simulink model "PEArray_co_sim"  (R2021a)
settings: Solver=VariableStepAuto  StartTime=0.0  StopTime=15  RelTol=1e-3
undefined symbols (not defined in the file or in its folder): A, N
libraries: hdlBasic x164, xbsIndex_r4 x1, JTAGRuntimeCosim_r4 x1
(part 2 of 2)

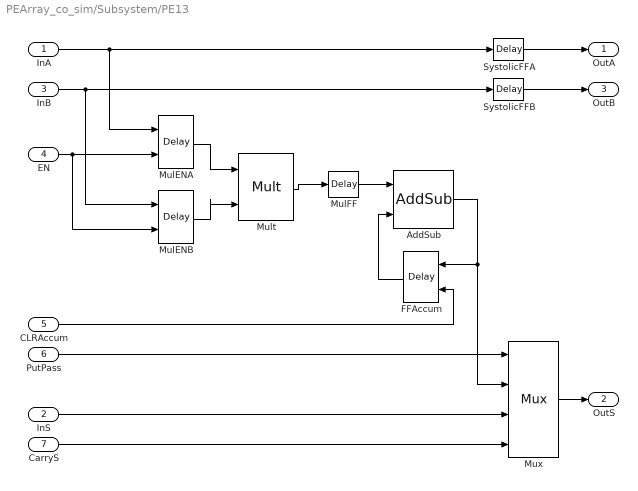
== system PEArray_co_sim/Subsystem/PE13 ==
  InA : Inport
  InS : Inport  Port=2
  InB : Inport  Port=3
  EN : Inport  Port=4
  CLRAccum : Inport  Port=5
  PutPass : Inport  Port=6
  CarryS : Inport  Port=7
  AddSub : hdlBasic/AddSub  mode=Addition  use_carryin=off  use_carryout=off  en=off  latency=0  precision=User Defined  arith_type="Signed  (2's comp)"  n_bits=16  bin_pt=10  quantization=Truncate  overflow=Wrap  use_behavioral_HDL=off  hw_selection=DSP48  pipelined=off  XmcBlockStatus=1  maskContainerNames=tabcontainer1  block_type=addsub  block_config=sysgen:Addsub_config
  FFAccum : hdlBasic/Delay  rst=on  en=off  latency=1  reg_retiming=off  XmcBlockStatus=1  maskContainerNames=group1  block_type=delay  block_config=sysgen:Delay_config
  MulENA : hdlBasic/Delay  rst=on  en=off  latency=1  reg_retiming=off  XmcBlockStatus=1  maskContainerNames=group1  block_type=delay  block_config=sysgen:Delay_config
  MulENB : hdlBasic/Delay  rst=on  en=off  latency=1  reg_retiming=off  XmcBlockStatus=1  maskContainerNames=group1  block_type=delay  block_config=sysgen:Delay_config
  MulFF : hdlBasic/Delay  rst=off  en=off  latency=1  reg_retiming=off  XmcBlockStatus=1  maskContainerNames=group1  block_type=delay  block_config=sysgen:Delay_config
  Mult : hdlBasic/Mult  precision=User Defined  arith_type="Signed  (2's comp)"  n_bits=16  bin_pt=10  quantization=Truncate  overflow=Wrap  en=off  latency=0  use_behavioral_HDL=off  opt=Speed  use_embedded=on  optimum_pipeline=off  pipeline=on  use_rpm=on  placement_style=Triangular  XmcBlockStatus=1  maskContainerNames=group1  block_type=mult  block_config=sysgen:Mult_config
  Mux : hdlBasic/Mux  inputs=2  en=on  latency=1  precision=Full  arith_type=Unsigned  n_bits=16  bin_pt=14  quantization=Truncate  overflow=Wrap  XmcBlockStatus=1  maskContainerNames=tabcontainer1  block_type=mux  block_config=sysgen:Mux_config
  SystolicFFA : hdlBasic/Delay  rst=off  en=off  latency=1  reg_retiming=off  XmcBlockStatus=1  maskContainerNames=group1  block_type=delay  block_config=sysgen:Delay_config
  SystolicFFB : hdlBasic/Delay  rst=off  en=off  latency=1  reg_retiming=off  XmcBlockStatus=1  maskContainerNames=group1  block_type=delay  block_config=sysgen:Delay_config
  OutA : Outport
  OutS : Outport  Port=2
  OutB : Outport  Port=3
  wires:
  Mult/1 -> MulFF/1
  MulFF/1 -> AddSub/1
  AddSub/1 -> Mux/2, FFAccum/1
  InB/1 -> MulENB/1, SystolicFFB/1
  InA/1 -> MulENA/1, SystolicFFA/1
  SystolicFFB/1 -> OutB/1
  SystolicFFA/1 -> OutA/1
  MulENA/1 -> Mult/1
  MulENB/1 -> Mult/2
  EN/1 -> MulENB/2, MulENA/2
  FFAccum/1 -> AddSub/2
  CLRAccum/1 -> FFAccum/2
  PutPass/1 -> Mux/1
  InS/1 -> Mux/3
  Mux/1 -> OutS/1
  CarryS/1 -> Mux/4

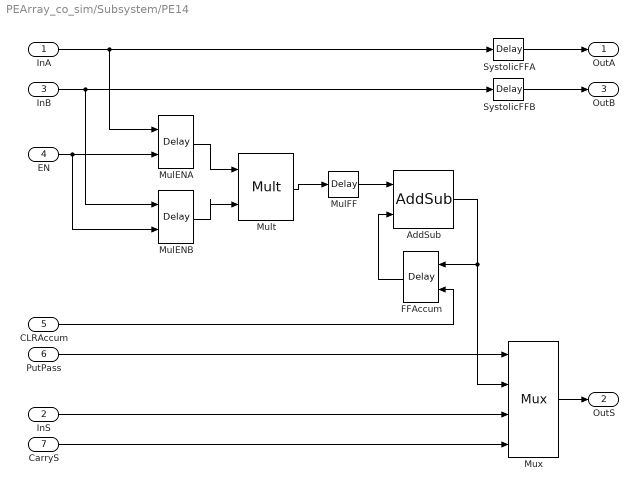
== system PEArray_co_sim/Subsystem/PE14 ==
  InA : Inport
  InS : Inport  Port=2
  InB : Inport  Port=3
  EN : Inport  Port=4
  CLRAccum : Inport  Port=5
  PutPass : Inport  Port=6
  CarryS : Inport  Port=7
  AddSub : hdlBasic/AddSub  mode=Addition  use_carryin=off  use_carryout=off  en=off  latency=0  precision=User Defined  arith_type="Signed  (2's comp)"  n_bits=16  bin_pt=10  quantization=Truncate  overflow=Wrap  use_behavioral_HDL=off  hw_selection=DSP48  pipelined=off  XmcBlockStatus=1  maskContainerNames=tabcontainer1  block_type=addsub  block_config=sysgen:Addsub_config
  FFAccum : hdlBasic/Delay  rst=on  en=off  latency=1  reg_retiming=off  XmcBlockStatus=1  maskContainerNames=group1  block_type=delay  block_config=sysgen:Delay_config
  MulENA : hdlBasic/Delay  rst=on  en=off  latency=1  reg_retiming=off  XmcBlockStatus=1  maskContainerNames=group1  block_type=delay  block_config=sysgen:Delay_config
  MulENB : hdlBasic/Delay  rst=on  en=off  latency=1  reg_retiming=off  XmcBlockStatus=1  maskContainerNames=group1  block_type=delay  block_config=sysgen:Delay_config
  MulFF : hdlBasic/Delay  rst=off  en=off  latency=1  reg_retiming=off  XmcBlockStatus=1  maskContainerNames=group1  block_type=delay  block_config=sysgen:Delay_config
  Mult : hdlBasic/Mult  precision=User Defined  arith_type="Signed  (2's comp)"  n_bits=16  bin_pt=10  quantization=Truncate  overflow=Wrap  en=off  latency=0  use_behavioral_HDL=off  opt=Speed  use_embedded=on  optimum_pipeline=off  pipeline=on  use_rpm=on  placement_style=Triangular  XmcBlockStatus=1  maskContainerNames=group1  block_type=mult  block_config=sysgen:Mult_config
  Mux : hdlBasic/Mux  inputs=2  en=on  latency=1  precision=Full  arith_type=Unsigned  n_bits=16  bin_pt=14  quantization=Truncate  overflow=Wrap  XmcBlockStatus=1  maskContainerNames=tabcontainer1  block_type=mux  block_config=sysgen:Mux_config
  SystolicFFA : hdlBasic/Delay  rst=off  en=off  latency=1  reg_retiming=off  XmcBlockStatus=1  maskContainerNames=group1  block_type=delay  block_config=sysgen:Delay_config
  SystolicFFB : hdlBasic/Delay  rst=off  en=off  latency=1  reg_retiming=off  XmcBlockStatus=1  maskContainerNames=group1  block_type=delay  block_config=sysgen:Delay_config
  OutA : Outport
  OutS : Outport  Port=2
  OutB : Outport  Port=3
  wires:
  Mult/1 -> MulFF/1
  MulFF/1 -> AddSub/1
  AddSub/1 -> Mux/2, FFAccum/1
  InB/1 -> MulENB/1, SystolicFFB/1
  InA/1 -> MulENA/1, SystolicFFA/1
  SystolicFFB/1 -> OutB/1
  SystolicFFA/1 -> OutA/1
  MulENA/1 -> Mult/1
  MulENB/1 -> Mult/2
  EN/1 -> MulENB/2, MulENA/2
  FFAccum/1 -> AddSub/2
  CLRAccum/1 -> FFAccum/2
  PutPass/1 -> Mux/1
  InS/1 -> Mux/3
  Mux/1 -> OutS/1
  CarryS/1 -> Mux/4

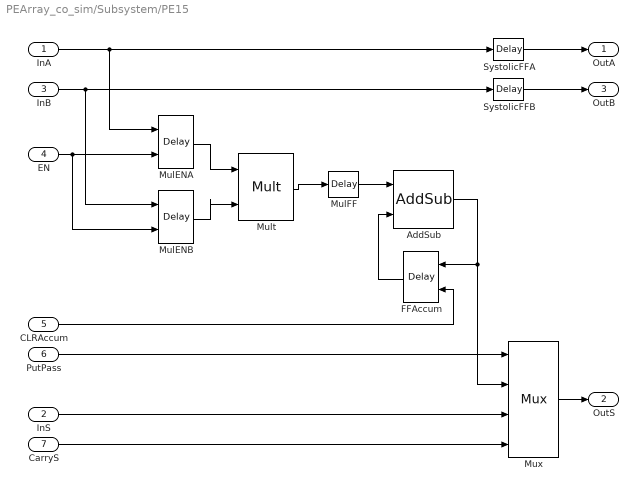
== system PEArray_co_sim/Subsystem/PE15 ==
  InA : Inport
  InS : Inport  Port=2
  InB : Inport  Port=3
  EN : Inport  Port=4
  CLRAccum : Inport  Port=5
  PutPass : Inport  Port=6
  CarryS : Inport  Port=7
  AddSub : hdlBasic/AddSub  mode=Addition  use_carryin=off  use_carryout=off  en=off  latency=0  precision=User Defined  arith_type="Signed  (2's comp)"  n_bits=16  bin_pt=10  quantization=Truncate  overflow=Wrap  use_behavioral_HDL=off  hw_selection=DSP48  pipelined=off  XmcBlockStatus=1  maskContainerNames=tabcontainer1  block_type=addsub  block_config=sysgen:Addsub_config
  FFAccum : hdlBasic/Delay  rst=on  en=off  latency=1  reg_retiming=off  XmcBlockStatus=1  maskContainerNames=group1  block_type=delay  block_config=sysgen:Delay_config
  MulENA : hdlBasic/Delay  rst=on  en=off  latency=1  reg_retiming=off  XmcBlockStatus=1  maskContainerNames=group1  block_type=delay  block_config=sysgen:Delay_config
  MulENB : hdlBasic/Delay  rst=on  en=off  latency=1  reg_retiming=off  XmcBlockStatus=1  maskContainerNames=group1  block_type=delay  block_config=sysgen:Delay_config
  MulFF : hdlBasic/Delay  rst=off  en=off  latency=1  reg_retiming=off  XmcBlockStatus=1  maskContainerNames=group1  block_type=delay  block_config=sysgen:Delay_config
  Mult : hdlBasic/Mult  precision=User Defined  arith_type="Signed  (2's comp)"  n_bits=16  bin_pt=10  quantization=Truncate  overflow=Wrap  en=off  latency=0  use_behavioral_HDL=off  opt=Speed  use_embedded=on  optimum_pipeline=off  pipeline=on  use_rpm=on  placement_style=Triangular  XmcBlockStatus=1  maskContainerNames=group1  block_type=mult  block_config=sysgen:Mult_config
  Mux : hdlBasic/Mux  inputs=2  en=on  latency=1  precision=Full  arith_type=Unsigned  n_bits=16  bin_pt=14  quantization=Truncate  overflow=Wrap  XmcBlockStatus=1  maskContainerNames=tabcontainer1  block_type=mux  block_config=sysgen:Mux_config
  SystolicFFA : hdlBasic/Delay  rst=off  en=off  latency=1  reg_retiming=off  XmcBlockStatus=1  maskContainerNames=group1  block_type=delay  block_config=sysgen:Delay_config
  SystolicFFB : hdlBasic/Delay  rst=off  en=off  latency=1  reg_retiming=off  XmcBlockStatus=1  maskContainerNames=group1  block_type=delay  block_config=sysgen:Delay_config
  OutA : Outport
  OutS : Outport  Port=2
  OutB : Outport  Port=3
  wires:
  Mult/1 -> MulFF/1
  MulFF/1 -> AddSub/1
  AddSub/1 -> Mux/2, FFAccum/1
  InB/1 -> MulENB/1, SystolicFFB/1
  InA/1 -> MulENA/1, SystolicFFA/1
  SystolicFFB/1 -> OutB/1
  SystolicFFA/1 -> OutA/1
  MulENA/1 -> Mult/1
  MulENB/1 -> Mult/2
  EN/1 -> MulENB/2, MulENA/2
  FFAccum/1 -> AddSub/2
  CLRAccum/1 -> FFAccum/2
  PutPass/1 -> Mux/1
  InS/1 -> Mux/3
  Mux/1 -> OutS/1
  CarryS/1 -> Mux/4

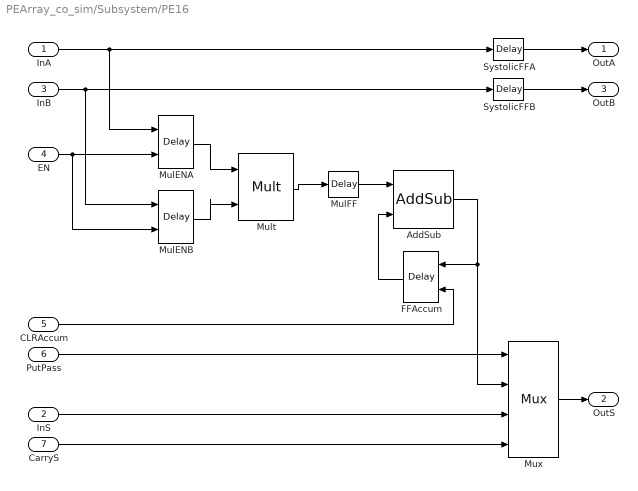
== system PEArray_co_sim/Subsystem/PE16 ==
  InA : Inport
  InS : Inport  Port=2
  InB : Inport  Port=3
  EN : Inport  Port=4
  CLRAccum : Inport  Port=5
  PutPass : Inport  Port=6
  CarryS : Inport  Port=7
  AddSub : hdlBasic/AddSub  mode=Addition  use_carryin=off  use_carryout=off  en=off  latency=0  precision=User Defined  arith_type="Signed  (2's comp)"  n_bits=16  bin_pt=10  quantization=Truncate  overflow=Wrap  use_behavioral_HDL=off  hw_selection=DSP48  pipelined=off  XmcBlockStatus=1  maskContainerNames=tabcontainer1  block_type=addsub  block_config=sysgen:Addsub_config
  FFAccum : hdlBasic/Delay  rst=on  en=off  latency=1  reg_retiming=off  XmcBlockStatus=1  maskContainerNames=group1  block_type=delay  block_config=sysgen:Delay_config
  MulENA : hdlBasic/Delay  rst=on  en=off  latency=1  reg_retiming=off  XmcBlockStatus=1  maskContainerNames=group1  block_type=delay  block_config=sysgen:Delay_config
  MulENB : hdlBasic/Delay  rst=on  en=off  latency=1  reg_retiming=off  XmcBlockStatus=1  maskContainerNames=group1  block_type=delay  block_config=sysgen:Delay_config
  MulFF : hdlBasic/Delay  rst=off  en=off  latency=1  reg_retiming=off  XmcBlockStatus=1  maskContainerNames=group1  block_type=delay  block_config=sysgen:Delay_config
  Mult : hdlBasic/Mult  precision=User Defined  arith_type="Signed  (2's comp)"  n_bits=16  bin_pt=10  quantization=Truncate  overflow=Wrap  en=off  latency=0  use_behavioral_HDL=off  opt=Speed  use_embedded=on  optimum_pipeline=off  pipeline=on  use_rpm=on  placement_style=Triangular  XmcBlockStatus=1  maskContainerNames=group1  block_type=mult  block_config=sysgen:Mult_config
  Mux : hdlBasic/Mux  inputs=2  en=on  latency=1  precision=Full  arith_type=Unsigned  n_bits=16  bin_pt=14  quantization=Truncate  overflow=Wrap  XmcBlockStatus=1  maskContainerNames=tabcontainer1  block_type=mux  block_config=sysgen:Mux_config
  SystolicFFA : hdlBasic/Delay  rst=off  en=off  latency=1  reg_retiming=off  XmcBlockStatus=1  maskContainerNames=group1  block_type=delay  block_config=sysgen:Delay_config
  SystolicFFB : hdlBasic/Delay  rst=off  en=off  latency=1  reg_retiming=off  XmcBlockStatus=1  maskContainerNames=group1  block_type=delay  block_config=sysgen:Delay_config
  OutA : Outport
  OutS : Outport  Port=2
  OutB : Outport  Port=3
  wires:
  Mult/1 -> MulFF/1
  MulFF/1 -> AddSub/1
  AddSub/1 -> Mux/2, FFAccum/1
  InB/1 -> MulENB/1, SystolicFFB/1
  InA/1 -> MulENA/1, SystolicFFA/1
  SystolicFFB/1 -> OutB/1
  SystolicFFA/1 -> OutA/1
  MulENA/1 -> Mult/1
  MulENB/1 -> Mult/2
  EN/1 -> MulENB/2, MulENA/2
  FFAccum/1 -> AddSub/2
  CLRAccum/1 -> FFAccum/2
  PutPass/1 -> Mux/1
  InS/1 -> Mux/3
  Mux/1 -> OutS/1
  CarryS/1 -> Mux/4

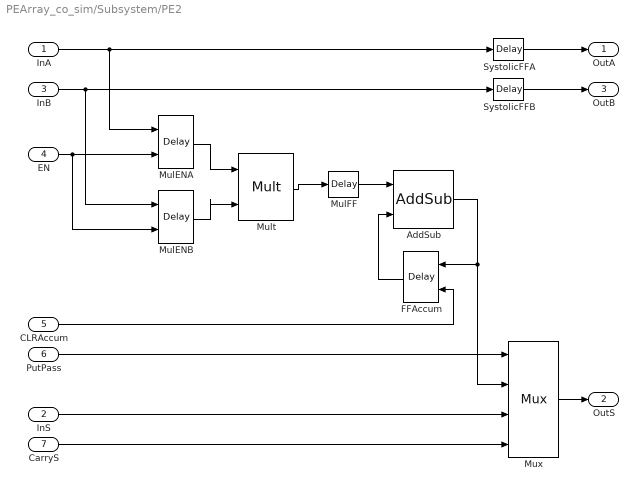
== system PEArray_co_sim/Subsystem/PE2 ==
  InA : Inport
  InS : Inport  Port=2
  InB : Inport  Port=3
  EN : Inport  Port=4
  CLRAccum : Inport  Port=5
  PutPass : Inport  Port=6
  CarryS : Inport  Port=7
  AddSub : hdlBasic/AddSub  mode=Addition  use_carryin=off  use_carryout=off  en=off  latency=0  precision=User Defined  arith_type="Signed  (2's comp)"  n_bits=16  bin_pt=10  quantization=Truncate  overflow=Wrap  use_behavioral_HDL=off  hw_selection=DSP48  pipelined=off  XmcBlockStatus=1  maskContainerNames=tabcontainer1  block_type=addsub  block_config=sysgen:Addsub_config
  FFAccum : hdlBasic/Delay  rst=on  en=off  latency=1  reg_retiming=off  XmcBlockStatus=1  maskContainerNames=group1  block_type=delay  block_config=sysgen:Delay_config
  MulENA : hdlBasic/Delay  rst=on  en=off  latency=1  reg_retiming=off  XmcBlockStatus=1  maskContainerNames=group1  block_type=delay  block_config=sysgen:Delay_config
  MulENB : hdlBasic/Delay  rst=on  en=off  latency=1  reg_retiming=off  XmcBlockStatus=1  maskContainerNames=group1  block_type=delay  block_config=sysgen:Delay_config
  MulFF : hdlBasic/Delay  rst=off  en=off  latency=1  reg_retiming=off  XmcBlockStatus=1  maskContainerNames=group1  block_type=delay  block_config=sysgen:Delay_config
  Mult : hdlBasic/Mult  precision=User Defined  arith_type="Signed  (2's comp)"  n_bits=16  bin_pt=10  quantization=Truncate  overflow=Wrap  en=off  latency=0  use_behavioral_HDL=off  opt=Speed  use_embedded=on  optimum_pipeline=off  pipeline=on  use_rpm=on  placement_style=Triangular  XmcBlockStatus=1  maskContainerNames=group1  block_type=mult  block_config=sysgen:Mult_config
  Mux : hdlBasic/Mux  inputs=2  en=on  latency=1  precision=Full  arith_type=Unsigned  n_bits=16  bin_pt=14  quantization=Truncate  overflow=Wrap  XmcBlockStatus=1  maskContainerNames=tabcontainer1  block_type=mux  block_config=sysgen:Mux_config
  SystolicFFA : hdlBasic/Delay  rst=off  en=off  latency=1  reg_retiming=off  XmcBlockStatus=1  maskContainerNames=group1  block_type=delay  block_config=sysgen:Delay_config
  SystolicFFB : hdlBasic/Delay  rst=off  en=off  latency=1  reg_retiming=off  XmcBlockStatus=1  maskContainerNames=group1  block_type=delay  block_config=sysgen:Delay_config
  OutA : Outport
  OutS : Outport  Port=2
  OutB : Outport  Port=3
  wires:
  Mult/1 -> MulFF/1
  MulFF/1 -> AddSub/1
  AddSub/1 -> Mux/2, FFAccum/1
  InB/1 -> MulENB/1, SystolicFFB/1
  InA/1 -> MulENA/1, SystolicFFA/1
  SystolicFFB/1 -> OutB/1
  SystolicFFA/1 -> OutA/1
  MulENA/1 -> Mult/1
  MulENB/1 -> Mult/2
  EN/1 -> MulENB/2, MulENA/2
  FFAccum/1 -> AddSub/2
  CLRAccum/1 -> FFAccum/2
  PutPass/1 -> Mux/1
  InS/1 -> Mux/3
  Mux/1 -> OutS/1
  CarryS/1 -> Mux/4

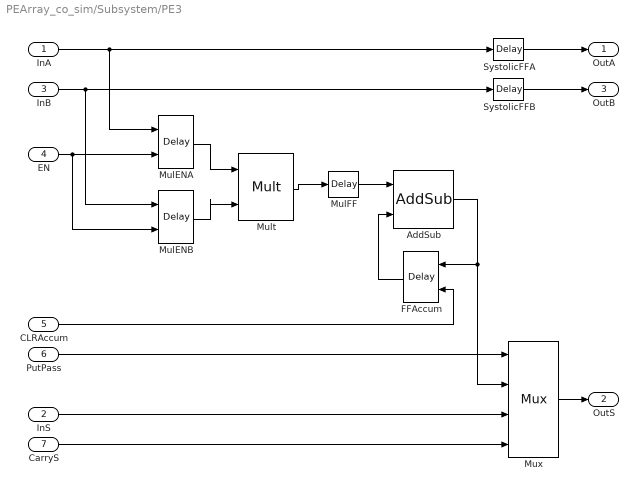
== system PEArray_co_sim/Subsystem/PE3 ==
  InA : Inport
  InS : Inport  Port=2
  InB : Inport  Port=3
  EN : Inport  Port=4
  CLRAccum : Inport  Port=5
  PutPass : Inport  Port=6
  CarryS : Inport  Port=7
  AddSub : hdlBasic/AddSub  mode=Addition  use_carryin=off  use_carryout=off  en=off  latency=0  precision=User Defined  arith_type="Signed  (2's comp)"  n_bits=16  bin_pt=10  quantization=Truncate  overflow=Wrap  use_behavioral_HDL=off  hw_selection=DSP48  pipelined=off  XmcBlockStatus=1  maskContainerNames=tabcontainer1  block_type=addsub  block_config=sysgen:Addsub_config
  FFAccum : hdlBasic/Delay  rst=on  en=off  latency=1  reg_retiming=off  XmcBlockStatus=1  maskContainerNames=group1  block_type=delay  block_config=sysgen:Delay_config
  MulENA : hdlBasic/Delay  rst=on  en=off  latency=1  reg_retiming=off  XmcBlockStatus=1  maskContainerNames=group1  block_type=delay  block_config=sysgen:Delay_config
  MulENB : hdlBasic/Delay  rst=on  en=off  latency=1  reg_retiming=off  XmcBlockStatus=1  maskContainerNames=group1  block_type=delay  block_config=sysgen:Delay_config
  MulFF : hdlBasic/Delay  rst=off  en=off  latency=1  reg_retiming=off  XmcBlockStatus=1  maskContainerNames=group1  block_type=delay  block_config=sysgen:Delay_config
  Mult : hdlBasic/Mult  precision=User Defined  arith_type="Signed  (2's comp)"  n_bits=16  bin_pt=10  quantization=Truncate  overflow=Wrap  en=off  latency=0  use_behavioral_HDL=off  opt=Speed  use_embedded=on  optimum_pipeline=off  pipeline=on  use_rpm=on  placement_style=Triangular  XmcBlockStatus=1  maskContainerNames=group1  block_type=mult  block_config=sysgen:Mult_config
  Mux : hdlBasic/Mux  inputs=2  en=on  latency=1  precision=Full  arith_type=Unsigned  n_bits=16  bin_pt=14  quantization=Truncate  overflow=Wrap  XmcBlockStatus=1  maskContainerNames=tabcontainer1  block_type=mux  block_config=sysgen:Mux_config
  SystolicFFA : hdlBasic/Delay  rst=off  en=off  latency=1  reg_retiming=off  XmcBlockStatus=1  maskContainerNames=group1  block_type=delay  block_config=sysgen:Delay_config
  SystolicFFB : hdlBasic/Delay  rst=off  en=off  latency=1  reg_retiming=off  XmcBlockStatus=1  maskContainerNames=group1  block_type=delay  block_config=sysgen:Delay_config
  OutA : Outport
  OutS : Outport  Port=2
  OutB : Outport  Port=3
  wires:
  Mult/1 -> MulFF/1
  MulFF/1 -> AddSub/1
  AddSub/1 -> Mux/2, FFAccum/1
  InB/1 -> MulENB/1, SystolicFFB/1
  InA/1 -> MulENA/1, SystolicFFA/1
  SystolicFFB/1 -> OutB/1
  SystolicFFA/1 -> OutA/1
  MulENA/1 -> Mult/1
  MulENB/1 -> Mult/2
  EN/1 -> MulENB/2, MulENA/2
  FFAccum/1 -> AddSub/2
  CLRAccum/1 -> FFAccum/2
  PutPass/1 -> Mux/1
  InS/1 -> Mux/3
  Mux/1 -> OutS/1
  CarryS/1 -> Mux/4

== system PEArray_co_sim/Subsystem/PE4 ==
  InA : Inport
  InS : Inport  Port=2
  InB : Inport  Port=3
  EN : Inport  Port=4
  CLRAccum : Inport  Port=5
  PutPass : Inport  Port=6
  CarryS : Inport  Port=7
  AddSub : hdlBasic/AddSub  mode=Addition  use_carryin=off  use_carryout=off  en=off  latency=0  precision=User Defined  arith_type="Signed  (2's comp)"  n_bits=16  bin_pt=10  quantization=Truncate  overflow=Wrap  use_behavioral_HDL=off  hw_selection=DSP48  pipelined=off  XmcBlockStatus=1  maskContainerNames=tabcontainer1  block_type=addsub  block_config=sysgen:Addsub_config
  FFAccum : hdlBasic/Delay  rst=on  en=off  latency=1  reg_retiming=off  XmcBlockStatus=1  maskContainerNames=group1  block_type=delay  block_config=sysgen:Delay_config
  MulENA : hdlBasic/Delay  rst=on  en=off  latency=1  reg_retiming=off  XmcBlockStatus=1  maskContainerNames=group1  block_type=delay  block_config=sysgen:Delay_config
  MulENB : hdlBasic/Delay  rst=on  en=off  latency=1  reg_retiming=off  XmcBlockStatus=1  maskContainerNames=group1  block_type=delay  block_config=sysgen:Delay_config
  MulFF : hdlBasic/Delay  rst=off  en=off  latency=1  reg_retiming=off  XmcBlockStatus=1  maskContainerNames=group1  block_type=delay  block_config=sysgen:Delay_config
  Mult : hdlBasic/Mult  precision=User Defined  arith_type="Signed  (2's comp)"  n_bits=16  bin_pt=10  quantization=Truncate  overflow=Wrap  en=off  latency=0  use_behavioral_HDL=off  opt=Speed  use_embedded=on  optimum_pipeline=off  pipeline=on  use_rpm=on  placement_style=Triangular  XmcBlockStatus=1  maskContainerNames=group1  block_type=mult  block_config=sysgen:Mult_config
  Mux : hdlBasic/Mux  inputs=2  en=on  latency=1  precision=Full  arith_type=Unsigned  n_bits=16  bin_pt=14  quantization=Truncate  overflow=Wrap  XmcBlockStatus=1  maskContainerNames=tabcontainer1  block_type=mux  block_config=sysgen:Mux_config
  SystolicFFA : hdlBasic/Delay  rst=off  en=off  latency=1  reg_retiming=off  XmcBlockStatus=1  maskContainerNames=group1  block_type=delay  block_config=sysgen:Delay_config
  SystolicFFB : hdlBasic/Delay  rst=off  en=off  latency=1  reg_retiming=off  XmcBlockStatus=1  maskContainerNames=group1  block_type=delay  block_config=sysgen:Delay_config
  OutA : Outport
  OutS : Outport  Port=2
  OutB : Outport  Port=3
  wires:
  Mult/1 -> MulFF/1
  MulFF/1 -> AddSub/1
  AddSub/1 -> Mux/2, FFAccum/1
  InB/1 -> MulENB/1, SystolicFFB/1
  InA/1 -> MulENA/1, SystolicFFA/1
  SystolicFFB/1 -> OutB/1
  SystolicFFA/1 -> OutA/1
  MulENA/1 -> Mult/1
  MulENB/1 -> Mult/2
  EN/1 -> MulENB/2, MulENA/2
  FFAccum/1 -> AddSub/2
  CLRAccum/1 -> FFAccum/2
  PutPass/1 -> Mux/1
  InS/1 -> Mux/3
  Mux/1 -> OutS/1
  CarryS/1 -> Mux/4

== system PEArray_co_sim/Subsystem/PE5 ==
  InA : Inport
  InS : Inport  Port=2
  InB : Inport  Port=3
  EN : Inport  Port=4
  CLRAccum : Inport  Port=5
  PutPass : Inport  Port=6
  CarryS : Inport  Port=7
  AddSub : hdlBasic/AddSub  mode=Addition  use_carryin=off  use_carryout=off  en=off  latency=0  precision=User Defined  arith_type="Signed  (2's comp)"  n_bits=16  bin_pt=10  quantization=Truncate  overflow=Wrap  use_behavioral_HDL=off  hw_selection=DSP48  pipelined=off  XmcBlockStatus=1  maskContainerNames=tabcontainer1  block_type=addsub  block_config=sysgen:Addsub_config
  FFAccum : hdlBasic/Delay  rst=on  en=off  latency=1  reg_retiming=off  XmcBlockStatus=1  maskContainerNames=group1  block_type=delay  block_config=sysgen:Delay_config
  MulENA : hdlBasic/Delay  rst=on  en=off  latency=1  reg_retiming=off  XmcBlockStatus=1  maskContainerNames=group1  block_type=delay  block_config=sysgen:Delay_config
  MulENB : hdlBasic/Delay  rst=on  en=off  latency=1  reg_retiming=off  XmcBlockStatus=1  maskContainerNames=group1  block_type=delay  block_config=sysgen:Delay_config
  MulFF : hdlBasic/Delay  rst=off  en=off  latency=1  reg_retiming=off  XmcBlockStatus=1  maskContainerNames=group1  block_type=delay  block_config=sysgen:Delay_config
  Mult : hdlBasic/Mult  precision=User Defined  arith_type="Signed  (2's comp)"  n_bits=16  bin_pt=10  quantization=Truncate  overflow=Wrap  en=off  latency=0  use_behavioral_HDL=off  opt=Speed  use_embedded=on  optimum_pipeline=off  pipeline=on  use_rpm=on  placement_style=Triangular  XmcBlockStatus=1  maskContainerNames=group1  block_type=mult  block_config=sysgen:Mult_config
  Mux : hdlBasic/Mux  inputs=2  en=on  latency=1  precision=Full  arith_type=Unsigned  n_bits=16  bin_pt=14  quantization=Truncate  overflow=Wrap  XmcBlockStatus=1  maskContainerNames=tabcontainer1  block_type=mux  block_config=sysgen:Mux_config
  SystolicFFA : hdlBasic/Delay  rst=off  en=off  latency=1  reg_retiming=off  XmcBlockStatus=1  maskContainerNames=group1  block_type=delay  block_config=sysgen:Delay_config
  SystolicFFB : hdlBasic/Delay  rst=off  en=off  latency=1  reg_retiming=off  XmcBlockStatus=1  maskContainerNames=group1  block_type=delay  block_config=sysgen:Delay_config
  OutA : Outport
  OutS : Outport  Port=2
  OutB : Outport  Port=3
  wires:
  Mult/1 -> MulFF/1
  MulFF/1 -> AddSub/1
  AddSub/1 -> Mux/2, FFAccum/1
  InB/1 -> MulENB/1, SystolicFFB/1
  InA/1 -> MulENA/1, SystolicFFA/1
  SystolicFFB/1 -> OutB/1
  SystolicFFA/1 -> OutA/1
  MulENA/1 -> Mult/1
  MulENB/1 -> Mult/2
  EN/1 -> MulENB/2, MulENA/2
  FFAccum/1 -> AddSub/2
  CLRAccum/1 -> FFAccum/2
  PutPass/1 -> Mux/1
  InS/1 -> Mux/3
  Mux/1 -> OutS/1
  CarryS/1 -> Mux/4

== system PEArray_co_sim/Subsystem/PE6 ==
  InA : Inport
  InS : Inport  Port=2
  InB : Inport  Port=3
  EN : Inport  Port=4
  CLRAccum : Inport  Port=5
  PutPass : Inport  Port=6
  CarryS : Inport  Port=7
  AddSub : hdlBasic/AddSub  mode=Addition  use_carryin=off  use_carryout=off  en=off  latency=0  precision=User Defined  arith_type="Signed  (2's comp)"  n_bits=16  bin_pt=10  quantization=Truncate  overflow=Wrap  use_behavioral_HDL=off  hw_selection=DSP48  pipelined=off  XmcBlockStatus=1  maskContainerNames=tabcontainer1  block_type=addsub  block_config=sysgen:Addsub_config
  FFAccum : hdlBasic/Delay  rst=on  en=off  latency=1  reg_retiming=off  XmcBlockStatus=1  maskContainerNames=group1  block_type=delay  block_config=sysgen:Delay_config
  MulENA : hdlBasic/Delay  rst=on  en=off  latency=1  reg_retiming=off  XmcBlockStatus=1  maskContainerNames=group1  block_type=delay  block_config=sysgen:Delay_config
  MulENB : hdlBasic/Delay  rst=on  en=off  latency=1  reg_retiming=off  XmcBlockStatus=1  maskContainerNames=group1  block_type=delay  block_config=sysgen:Delay_config
  MulFF : hdlBasic/Delay  rst=off  en=off  latency=1  reg_retiming=off  XmcBlockStatus=1  maskContainerNames=group1  block_type=delay  block_config=sysgen:Delay_config
  Mult : hdlBasic/Mult  precision=User Defined  arith_type="Signed  (2's comp)"  n_bits=16  bin_pt=10  quantization=Truncate  overflow=Wrap  en=off  latency=0  use_behavioral_HDL=off  opt=Speed  use_embedded=on  optimum_pipeline=off  pipeline=on  use_rpm=on  placement_style=Triangular  XmcBlockStatus=1  maskContainerNames=group1  block_type=mult  block_config=sysgen:Mult_config
  Mux : hdlBasic/Mux  inputs=2  en=on  latency=1  precision=Full  arith_type=Unsigned  n_bits=16  bin_pt=14  quantization=Truncate  overflow=Wrap  XmcBlockStatus=1  maskContainerNames=tabcontainer1  block_type=mux  block_config=sysgen:Mux_config
  SystolicFFA : hdlBasic/Delay  rst=off  en=off  latency=1  reg_retiming=off  XmcBlockStatus=1  maskContainerNames=group1  block_type=delay  block_config=sysgen:Delay_config
  SystolicFFB : hdlBasic/Delay  rst=off  en=off  latency=1  reg_retiming=off  XmcBlockStatus=1  maskContainerNames=group1  block_type=delay  block_config=sysgen:Delay_config
  OutA : Outport
  OutS : Outport  Port=2
  OutB : Outport  Port=3
  wires:
  Mult/1 -> MulFF/1
  MulFF/1 -> AddSub/1
  AddSub/1 -> Mux/2, FFAccum/1
  InB/1 -> MulENB/1, SystolicFFB/1
  InA/1 -> MulENA/1, SystolicFFA/1
  SystolicFFB/1 -> OutB/1
  SystolicFFA/1 -> OutA/1
  MulENA/1 -> Mult/1
  MulENB/1 -> Mult/2
  EN/1 -> MulENB/2, MulENA/2
  FFAccum/1 -> AddSub/2
  CLRAccum/1 -> FFAccum/2
  PutPass/1 -> Mux/1
  InS/1 -> Mux/3
  Mux/1 -> OutS/1
  CarryS/1 -> Mux/4

== system PEArray_co_sim/Subsystem/PE7 ==
  InA : Inport
  InS : Inport  Port=2
  InB : Inport  Port=3
  EN : Inport  Port=4
  CLRAccum : Inport  Port=5
  PutPass : Inport  Port=6
  CarryS : Inport  Port=7
  AddSub : hdlBasic/AddSub  mode=Addition  use_carryin=off  use_carryout=off  en=off  latency=0  precision=User Defined  arith_type="Signed  (2's comp)"  n_bits=16  bin_pt=10  quantization=Truncate  overflow=Wrap  use_behavioral_HDL=off  hw_selection=DSP48  pipelined=off  XmcBlockStatus=1  maskContainerNames=tabcontainer1  block_type=addsub  block_config=sysgen:Addsub_config
  FFAccum : hdlBasic/Delay  rst=on  en=off  latency=1  reg_retiming=off  XmcBlockStatus=1  maskContainerNames=group1  block_type=delay  block_config=sysgen:Delay_config
  MulENA : hdlBasic/Delay  rst=on  en=off  latency=1  reg_retiming=off  XmcBlockStatus=1  maskContainerNames=group1  block_type=delay  block_config=sysgen:Delay_config
  MulENB : hdlBasic/Delay  rst=on  en=off  latency=1  reg_retiming=off  XmcBlockStatus=1  maskContainerNames=group1  block_type=delay  block_config=sysgen:Delay_config
  MulFF : hdlBasic/Delay  rst=off  en=off  latency=1  reg_retiming=off  XmcBlockStatus=1  maskContainerNames=group1  block_type=delay  block_config=sysgen:Delay_config
  Mult : hdlBasic/Mult  precision=User Defined  arith_type="Signed  (2's comp)"  n_bits=16  bin_pt=10  quantization=Truncate  overflow=Wrap  en=off  latency=0  use_behavioral_HDL=off  opt=Speed  use_embedded=on  optimum_pipeline=off  pipeline=on  use_rpm=on  placement_style=Triangular  XmcBlockStatus=1  maskContainerNames=group1  block_type=mult  block_config=sysgen:Mult_config
  Mux : hdlBasic/Mux  inputs=2  en=on  latency=1  precision=Full  arith_type=Unsigned  n_bits=16  bin_pt=14  quantization=Truncate  overflow=Wrap  XmcBlockStatus=1  maskContainerNames=tabcontainer1  block_type=mux  block_config=sysgen:Mux_config
  SystolicFFA : hdlBasic/Delay  rst=off  en=off  latency=1  reg_retiming=off  XmcBlockStatus=1  maskContainerNames=group1  block_type=delay  block_config=sysgen:Delay_config
  SystolicFFB : hdlBasic/Delay  rst=off  en=off  latency=1  reg_retiming=off  XmcBlockStatus=1  maskContainerNames=group1  block_type=delay  block_config=sysgen:Delay_config
  OutA : Outport
  OutS : Outport  Port=2
  OutB : Outport  Port=3
  wires:
  Mult/1 -> MulFF/1
  MulFF/1 -> AddSub/1
  AddSub/1 -> Mux/2, FFAccum/1
  InB/1 -> MulENB/1, SystolicFFB/1
  InA/1 -> MulENA/1, SystolicFFA/1
  SystolicFFB/1 -> OutB/1
  SystolicFFA/1 -> OutA/1
  MulENA/1 -> Mult/1
  MulENB/1 -> Mult/2
  EN/1 -> MulENB/2, MulENA/2
  FFAccum/1 -> AddSub/2
  CLRAccum/1 -> FFAccum/2
  PutPass/1 -> Mux/1
  InS/1 -> Mux/3
  Mux/1 -> OutS/1
  CarryS/1 -> Mux/4

== system PEArray_co_sim/Subsystem/PE8 ==
  InA : Inport
  InS : Inport  Port=2
  InB : Inport  Port=3
  EN : Inport  Port=4
  CLRAccum : Inport  Port=5
  PutPass : Inport  Port=6
  CarryS : Inport  Port=7
  AddSub : hdlBasic/AddSub  mode=Addition  use_carryin=off  use_carryout=off  en=off  latency=0  precision=User Defined  arith_type="Signed  (2's comp)"  n_bits=16  bin_pt=10  quantization=Truncate  overflow=Wrap  use_behavioral_HDL=off  hw_selection=DSP48  pipelined=off  XmcBlockStatus=1  maskContainerNames=tabcontainer1  block_type=addsub  block_config=sysgen:Addsub_config
  FFAccum : hdlBasic/Delay  rst=on  en=off  latency=1  reg_retiming=off  XmcBlockStatus=1  maskContainerNames=group1  block_type=delay  block_config=sysgen:Delay_config
  MulENA : hdlBasic/Delay  rst=on  en=off  latency=1  reg_retiming=off  XmcBlockStatus=1  maskContainerNames=group1  block_type=delay  block_config=sysgen:Delay_config
  MulENB : hdlBasic/Delay  rst=on  en=off  latency=1  reg_retiming=off  XmcBlockStatus=1  maskContainerNames=group1  block_type=delay  block_config=sysgen:Delay_config
  MulFF : hdlBasic/Delay  rst=off  en=off  latency=1  reg_retiming=off  XmcBlockStatus=1  maskContainerNames=group1  block_type=delay  block_config=sysgen:Delay_config
  Mult : hdlBasic/Mult  precision=User Defined  arith_type="Signed  (2's comp)"  n_bits=16  bin_pt=10  quantization=Truncate  overflow=Wrap  en=off  latency=0  use_behavioral_HDL=off  opt=Speed  use_embedded=on  optimum_pipeline=off  pipeline=on  use_rpm=on  placement_style=Triangular  XmcBlockStatus=1  maskContainerNames=group1  block_type=mult  block_config=sysgen:Mult_config
  Mux : hdlBasic/Mux  inputs=2  en=on  latency=1  precision=Full  arith_type=Unsigned  n_bits=16  bin_pt=14  quantization=Truncate  overflow=Wrap  XmcBlockStatus=1  maskContainerNames=tabcontainer1  block_type=mux  block_config=sysgen:Mux_config
  SystolicFFA : hdlBasic/Delay  rst=off  en=off  latency=1  reg_retiming=off  XmcBlockStatus=1  maskContainerNames=group1  block_type=delay  block_config=sysgen:Delay_config
  SystolicFFB : hdlBasic/Delay  rst=off  en=off  latency=1  reg_retiming=off  XmcBlockStatus=1  maskContainerNames=group1  block_type=delay  block_config=sysgen:Delay_config
  OutA : Outport
  OutS : Outport  Port=2
  OutB : Outport  Port=3
  wires:
  Mult/1 -> MulFF/1
  MulFF/1 -> AddSub/1
  AddSub/1 -> Mux/2, FFAccum/1
  InB/1 -> MulENB/1, SystolicFFB/1
  InA/1 -> MulENA/1, SystolicFFA/1
  SystolicFFB/1 -> OutB/1
  SystolicFFA/1 -> OutA/1
  MulENA/1 -> Mult/1
  MulENB/1 -> Mult/2
  EN/1 -> MulENB/2, MulENA/2
  FFAccum/1 -> AddSub/2
  CLRAccum/1 -> FFAccum/2
  PutPass/1 -> Mux/1
  InS/1 -> Mux/3
  Mux/1 -> OutS/1
  CarryS/1 -> Mux/4

== system PEArray_co_sim/Subsystem/PE9 ==
  InA : Inport
  InS : Inport  Port=2
  InB : Inport  Port=3
  EN : Inport  Port=4
  CLRAccum : Inport  Port=5
  PutPass : Inport  Port=6
  CarryS : Inport  Port=7
  AddSub : hdlBasic/AddSub  mode=Addition  use_carryin=off  use_carryout=off  en=off  latency=0  precision=User Defined  arith_type="Signed  (2's comp)"  n_bits=16  bin_pt=10  quantization=Truncate  overflow=Wrap  use_behavioral_HDL=off  hw_selection=DSP48  pipelined=off  XmcBlockStatus=1  maskContainerNames=tabcontainer1  block_type=addsub  block_config=sysgen:Addsub_config
  FFAccum : hdlBasic/Delay  rst=on  en=off  latency=1  reg_retiming=off  XmcBlockStatus=1  maskContainerNames=group1  block_type=delay  block_config=sysgen:Delay_config
  MulENA : hdlBasic/Delay  rst=on  en=off  latency=1  reg_retiming=off  XmcBlockStatus=1  maskContainerNames=group1  block_type=delay  block_config=sysgen:Delay_config
  MulENB : hdlBasic/Delay  rst=on  en=off  latency=1  reg_retiming=off  XmcBlockStatus=1  maskContainerNames=group1  block_type=delay  block_config=sysgen:Delay_config
  MulFF : hdlBasic/Delay  rst=off  en=off  latency=1  reg_retiming=off  XmcBlockStatus=1  maskContainerNames=group1  block_type=delay  block_config=sysgen:Delay_config
  Mult : hdlBasic/Mult  precision=User Defined  arith_type="Signed  (2's comp)"  n_bits=16  bin_pt=10  quantization=Truncate  overflow=Wrap  en=off  latency=0  use_behavioral_HDL=off  opt=Speed  use_embedded=on  optimum_pipeline=off  pipeline=on  use_rpm=on  placement_style=Triangular  XmcBlockStatus=1  maskContainerNames=group1  block_type=mult  block_config=sysgen:Mult_config
  Mux : hdlBasic/Mux  inputs=2  en=on  latency=1  precision=Full  arith_type=Unsigned  n_bits=16  bin_pt=14  quantization=Truncate  overflow=Wrap  XmcBlockStatus=1  maskContainerNames=tabcontainer1  block_type=mux  block_config=sysgen:Mux_config
  SystolicFFA : hdlBasic/Delay  rst=off  en=off  latency=1  reg_retiming=off  XmcBlockStatus=1  maskContainerNames=group1  block_type=delay  block_config=sysgen:Delay_config
  SystolicFFB : hdlBasic/Delay  rst=off  en=off  latency=1  reg_retiming=off  XmcBlockStatus=1  maskContainerNames=group1  block_type=delay  block_config=sysgen:Delay_config
  OutA : Outport
  OutS : Outport  Port=2
  OutB : Outport  Port=3
  wires:
  Mult/1 -> MulFF/1
  MulFF/1 -> AddSub/1
  AddSub/1 -> Mux/2, FFAccum/1
  InB/1 -> MulENB/1, SystolicFFB/1
  InA/1 -> MulENA/1, SystolicFFA/1
  SystolicFFB/1 -> OutB/1
  SystolicFFA/1 -> OutA/1
  MulENA/1 -> Mult/1
  MulENB/1 -> Mult/2
  EN/1 -> MulENB/2, MulENA/2
  FFAccum/1 -> AddSub/2
  CLRAccum/1 -> FFAccum/2
  PutPass/1 -> Mux/1
  InS/1 -> Mux/3
  Mux/1 -> OutS/1
  CarryS/1 -> Mux/4
